simulink library "DoorRlsDriver"  (R2022a)
settings: Solver=VariableStepAuto  StartTime=0.0  StopTime=10.0  RelTol=1e-3
settings Model: Creator=DELL  LastModifiedBy=DELL

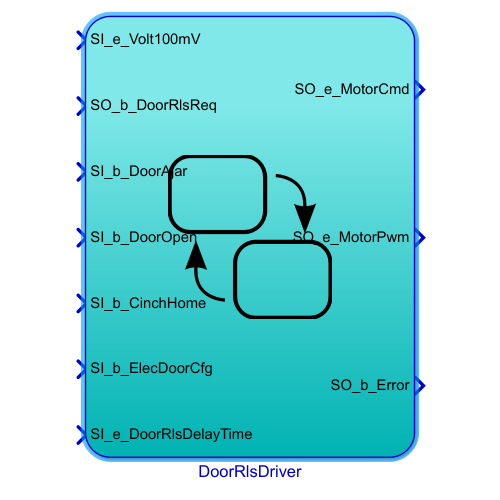
[thumbnail: Simulink's stored preview of the top-level diagram]
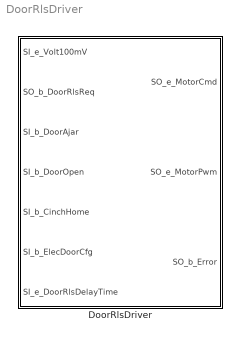
== system DoorRlsDriver ==
  DoorRlsDriver : Stateflow chart  TreatAsAtomicUnit=on

== stateflow chart DoorRlsDriver/DoorRlsDriver ==
  state PowerOn
    en:
    /* 上电释放电机执行一次复位 */
    SO_e_MotorCmd = 2;
    SO_e_MotorPwm = 100;
  note: SO_e_MotorCmd
      | 0: Stop
      | 1: Rls (A:1 B:0)
      | 2: Reset (A:0 B:1)
  state y = GetPwm(x) [function]
    (default) -> (junction 282) : {y = (x * 100 / SI_e_Volt100mV);}
        | /* 扩大100倍，浮点转整型 */
    (junction 282) -> (junction 286) [order 1] : [y > 100 || SI_e_Volt100mV == 0]
    (junction 282) -> (junction 288) [order 2]
    (junction 286) -> (junction 290) : {y = 100;}
    (junction 290) -> (junction 288)
    (junction 288) -> (junction 293)
  state Normal
    state NonElectricDoor
      state MainProgress [parallel]
        settings: executionOrder=1
        state Release
          en:
          SL_e_CycleCount = 0;
          state Delay
            /* 无框车门电释放延时 */
          state Step1_Ajar
            en:
            SO_e_MotorCmd = 1;
            SO_e_MotorPwm = GetPwm(105);
          state Check
            en:
            SO_e_MotorCmd = 0;
            SO_e_MotorPwm = 0;
          state Step2_Open
            state Idle
              en:
              SO_e_MotorCmd = 0;
              SO_e_MotorPwm = 0;
            state LastCheck
            (default) -> Normal.NonElectricDoor.MainProgress.Release.Step2_Open.Idle
            Normal.NonElectricDoor.MainProgress.Release.Step2_Open.Idle -> (junction 251) [order 1] : [before(270, tick) &&...
                | SI_b_DoorOpen == 1]
                | {SO_b_Error = 0;}
            (junction 251) -> (junction 242)
            Normal.NonElectricDoor.MainProgress.Release.Step2_Open.Idle -> Normal.NonElectricDoor.MainProgress.Release.Step2_Open.LastCheck [order 2] : [after(300, tick)]
            Normal.NonElectricDoor.MainProgress.Release.Step2_Open.LastCheck -> (junction 242)
          state Stall_Handle
            en:
            SO_e_MotorCmd = 1;
            SO_e_MotorPwm = 100;
            SL_e_CycleCount++;
          state Reset
            en:
            SO_e_MotorCmd = 2;
            SO_e_MotorPwm = GetPwm(70);
          (default) -> Normal.NonElectricDoor.MainProgress.Release.Delay
          Normal.NonElectricDoor.MainProgress.Release.Step1_Ajar -> Normal.NonElectricDoor.MainProgress.Release.Check : [after(30, tick)]
          Normal.NonElectricDoor.MainProgress.Release.Check -> Normal.NonElectricDoor.MainProgress.Release.Step2_Open [order 1] : [after(5, tick) &&...
              | SI_b_DoorAjar == 1]
          Normal.NonElectricDoor.MainProgress.Release.Delay -> Normal.NonElectricDoor.MainProgress.Release.Step1_Ajar : after(SL_e_DoorRlsDelayTime, tick)
          Normal.NonElectricDoor.MainProgress.Release.Stall_Handle -> Normal.NonElectricDoor.MainProgress.Release.Check : [after(30, tick)]
          Normal.NonElectricDoor.MainProgress.Release.Check -> Normal.NonElectricDoor.MainProgress.Release.Stall_Handle [order 2] : [after(5, tick) &&...
              | SI_b_DoorAjar == 0 &&...
              | SL_e_CycleCount < 3]
          Normal.NonElectricDoor.MainProgress.Release.Check -> Normal.NonElectricDoor.MainProgress.Release.Reset [order 3] : [after(5, tick) &&...
              | SI_b_DoorAjar == 0 &&...
              | SL_e_CycleCount >= 3]
              | {SO_b_Error = 1;}
          (junction 242) -> Normal.NonElectricDoor.MainProgress.Release.Reset
        state Idle
          en:
          SO_e_MotorCmd = 0;
          SO_e_MotorPwm = 0;
        (default) -> Normal.NonElectricDoor.MainProgress.Idle
        Normal.NonElectricDoor.MainProgress.Idle -> Normal.NonElectricDoor.MainProgress.Release : [SO_b_DoorRlsReq == 1]
            | {SL_e_DoorRlsDelayTime = SI_e_DoorRlsDelayTime;}
        Normal.NonElectricDoor.MainProgress.Release.Reset -> Normal.NonElectricDoor.MainProgress.Idle : [after(30, tick)]
    state ElectricDoor [commented out]
      state MainProgress [parallel] [commented out]
        state Release [commented out]
          en:
          SL_e_CycleCount = 0;
          state Step2_Open [commented out]
            state Idle [commented out]
              en:
              SO_e_MotorCmd = 0;
              SO_e_MotorPwm = 0;
            state Fail [commented out]
              en:
              SO_b_Error = 1;
            state LastCheck [commented out]
            state Ice_Break [commented out]
            state Fail1 [commented out]
              en:
              SO_b_Error = 1;
            state Success [commented out]
              en:
              SO_b_Error = 0;
            (default) -> Normal.ElectricDoor.MainProgress.Release.Step2_Open.Idle [commented out]
            Normal.ElectricDoor.MainProgress.Release.Step2_Open.Idle -> (junction 227) [commented out] : [before(270, tick) &&...
                | SI_b_DoorOpen == 1]
                | {SO_b_Error = 0;}
            (junction 227) -> (junction 219) [commented out]
            Normal.ElectricDoor.MainProgress.Release.Step2_Open.Idle -> Normal.ElectricDoor.MainProgress.Release.Step2_Open.LastCheck [commented out] : [after(300,tick)]
            Fail -> (junction 219) [commented out]
            Normal.ElectricDoor.MainProgress.Release.Step2_Open.LastCheck -> Fail [commented out] : [SI_b_CinchHome == 0]
            (junction 219) -> (junction 210) [commented out]
            Normal.ElectricDoor.MainProgress.Release.Step2_Open.LastCheck -> Ice_Break [commented out] : [SI_b_CinchHome == 1]
            Ice_Break -> Fail1 [commented out] : [after(600, tick) &&...
                | SI_b_CinchHome == 1]
            Fail1 -> (junction 210) [commented out]
            (junction 210) -> (junction 225) [commented out]
            Success -> (junction 225) [commented out]
            Ice_Break -> Success [commented out] : [before(600, tick) &&...
                | SI_b_CinchHome == 0]
          state Delay [commented out]
            /* 无框车门电释放延时 */
          state Step1_Ajar [commented out]
            en:
            SO_e_MotorCmd = 1;
            SO_e_MotorPwm = GetPwm(105);
          state Check [commented out]
            en:
            SO_e_MotorCmd = 0;
            SO_e_MotorPwm = 0;
          state Stall_Handle [commented out]
            en:
            SO_e_MotorCmd = 1;
            SO_e_MotorPwm = 100;
            SL_e_CycleCount++;
          state Reset [commented out]
            en:
            SO_e_MotorCmd = 2;
            SO_e_MotorPwm = GetPwm(70);
          (default) -> Normal.ElectricDoor.MainProgress.Release.Delay [commented out]
          Normal.ElectricDoor.MainProgress.Release.Step1_Ajar -> Normal.ElectricDoor.MainProgress.Release.Check [commented out] : [after(30, tick)]
          Normal.ElectricDoor.MainProgress.Release.Check -> Normal.ElectricDoor.MainProgress.Release.Step2_Open [commented out] : [after(5, tick) &&...
              | SI_b_DoorAjar == 1]
          Normal.ElectricDoor.MainProgress.Release.Delay -> Normal.ElectricDoor.MainProgress.Release.Step1_Ajar [commented out] : after(SL_e_DoorRlsDelayTime, tick)
          Normal.ElectricDoor.MainProgress.Release.Stall_Handle -> Normal.ElectricDoor.MainProgress.Release.Check [commented out] : [after(30, tick)]
          Normal.ElectricDoor.MainProgress.Release.Check -> Normal.ElectricDoor.MainProgress.Release.Stall_Handle [commented out] : [after(5, tick) &&...
              | SI_b_DoorAjar == 0 &&...
              | SL_e_CycleCount < 3]
          Normal.ElectricDoor.MainProgress.Release.Check -> Normal.ElectricDoor.MainProgress.Release.Reset [commented out] : [after(5, tick) &&...
              | SI_b_DoorAjar == 0 &&...
              | SL_e_CycleCount >= 3]
              | {SO_b_Error = 1;}
          (junction 225) -> Normal.ElectricDoor.MainProgress.Release.Reset [commented out]
        state Idle [commented out]
          en:
          SO_e_MotorCmd = 0;
          SO_e_MotorPwm = 0;
        (default) -> Normal.ElectricDoor.MainProgress.Idle [commented out]
        Normal.ElectricDoor.MainProgress.Idle -> Normal.ElectricDoor.MainProgress.Release [commented out] : [SO_b_DoorRlsReq == 1]
            | {SL_e_DoorRlsDelayTime = SI_e_DoorRlsDelayTime;}
        Normal.ElectricDoor.MainProgress.Release.Reset -> Normal.ElectricDoor.MainProgress.Idle [commented out] : [after(30, tick)]
    (default) -> NonElectricDoor
    ElectricDoor -> NonElectricDoor [commented out] : [SI_b_ElecDoorCfg == 0]
    NonElectricDoor -> ElectricDoor [commented out] : [SI_b_ElecDoorCfg == 1]
    (default) -> ElectricDoor [commented out] : [SI_b_ElecDoorCfg == 1]
        | /* 电动门 */
  (default) -> PowerOn
  PowerOn -> Normal : [after(30, tick)]
      | {SO_e_MotorCmd = 0;
      | SO_e_MotorPwm = 0;}
  data: x function_input double; y function_output double; SI_e_Volt100mV input uint8; SO_b_DoorRlsReq input boolean; SI_b_DoorAjar input boolean; SI_b_DoorOpen input boolean; SO_e_MotorCmd output uint8; SI_b_CinchHome input boolean; SI_b_ElecDoorCfg input boolean; SL_e_CycleCount local uint8; SO_e_MotorPwm output uint8; SO_b_Error output boolean; SI_e_DoorRlsDelayTime input uint8; SL_e_DoorRlsDelayTime local uint8
